simulink model "FFTT"  (R2015b)
settings: Solver=VariableStepAuto  StartTime=0.0  StopTime=10.0  RelTol=1e-3
undefined symbols (not defined in the file or in its folder): get
libraries: dspxfrm3 x1, dspsnks4 x1
settings Model: Creator=YogurtSuee  LastModifiedBy=YogurtSuee

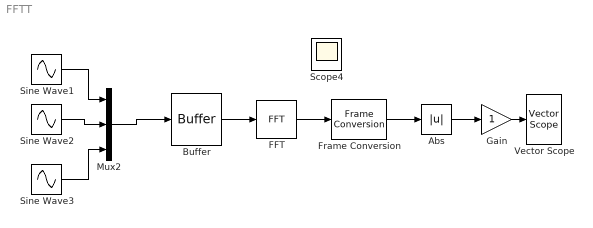
== system FFTT ==
  Abs : Abs
  Buffer : Buffer  N=256  TreatMby1Signals=One channel  OutputFrames=off
  FFT : dspxfrm3/FFT  FFTImplementation=Auto  CompMethod=Table lookup  TableOpt=NEW  TableOptActive=Speed  BitRevOrder=off  Normalize=off  InheritFFTLength=on  FFTLength=64  WrapInput=on  roundingMode=Floor  overflowMode=off  firstCoeffDataTypeStr=Inherit: Same word length as input  firstCoeffLastDataTypeStr=Inherit: Same word length as input  outputMin=[]  outputMax=[]
  Frame Conversion : FrameConversion  InheritSamplingMode=off
  Gain : Gain
  Mux2 : Mux  Inputs=3
  Scope4 : Scope
  Sine Wave1 : Sin  Amplitude=0.001  Frequency=0.1  SampleTime=0
  Sine Wave2 : Sin  Frequency=10  SampleTime=0
  Sine Wave3 : Sin  Amplitude=10  Frequency=100  SampleTime=0
  Vector Scope : dspsnks4/Vector Scope  ScopeProperties=on  Domain=Frequency  HorizSpan=1  DisplayProperties=off  AxisGrid=on  Memory=off  FrameNumber=on  AxisLegend=off  AxisZoom=on  OpenScopeAtSimStart=on  OpenScopeImmediately=off  FigPos=get(0,'defaultfigureposition')  AxisProperties=off  XUnits=Hertz  XRange=[0...Fs/2]  InheritXIncr=on  XIncr=1  XLabel=Time  XLimit=Auto  XMin=0  XMax=1  XStart=0  YUnits=Magnitude  YLabel=Amplitude  LineProperties=off  LineMarkers=+  XAxisParamsVer=6.9
      settings: YMin=-2  YMax=60
  wires:
  Buffer/1 -> FFT/1
  FFT/1 -> Frame Conversion/1
  Frame Conversion/1 -> Abs/1
  Abs/1 -> Gain/1
  Gain/1 -> Vector Scope/1
  Sine Wave1/1 -> Mux2/1
  Sine Wave2/1 -> Mux2/2
  Sine Wave3/1 -> Mux2/3
  Mux2/1 -> Buffer/1
